simulink model "DC_Motor_Current_Control"  (R2024b)
settings: Solver=FixedStepDiscrete  StartTime=0.0  StopTime=15  FixedStep=0.001  RelTol=1e-3  EnableMultiTasking=on
undefined symbols (not defined in the file or in its folder): dspblkCoreblockFVToolHelper, gcbh
libraries: simulink x4, arduinolib x4, slpidlib x1
settings Model: ExtModeTrigDuration=2  Creator=BU  LastModifiedBy=BU
settings SolverCC: AutoInsertRateTranBlk=on
settings OptimizationCC: EnhancedBackFolding=on  PassReuseOutputArgsAs=Individual arguments  ZeroExternalMemoryAtStartup=off  ZeroInternalMemoryAtStartup=off  MaxStackSize=64  OptimizeBlockOrder=speed  DifferentSizesBufferReuse=on  OptimizationCustomize=off  EfficientTunableParamExpr=on
settings DebuggingCC: ParameterTunabilityLossMsg=error
settings HardwareCC: ProdBitPerInt=16  ProdBitPerPointer=16  ProdBitPerSizeT=16  ProdBitPerPtrDiffT=16  ProdLargestAtomicFloat=None  ProdWordSize=8  ProdHWDeviceType=Atmel->AVR  UseEmbeddedCoderFeatures=off  UseSimulinkCoderFeatures=off
settings SFSimCC: MATLABDynamicMemAlloc=off
settings RTWCC: Description=Embedded Coder  SystemTargetFile=ert.tlc  HardwareBoard=Arduino Mega 2560  TemplateMakefile=ert_default_tmf  Toolchain=Arduino AVR  BuildConfiguration=Faster Runs
settings CodeAppCC: ForceParamTrailComments=on  IgnoreCustomStorageClasses=off  OperatorAnnotations=on  SimulinkDataObjDesc=on  SFDataObjDesc=on  MangleLength=10  InsertBlockDesc=on
settings ERTTargetCC: SupportContinuousTime=on  SupportNonInlinedSFcns=on  SupportVariableSizeSignals=on  ExtModeTransport=3  ExtModeStaticAlloc=on  ExtModeAutomaticAllocSize=off  ExtModeStaticAllocSize=2048  ExtModeMexFile=ext_xcp  ExtModeIntrfLevel=Level2 - Open  InlinedParameterPlacement=Hierarchical

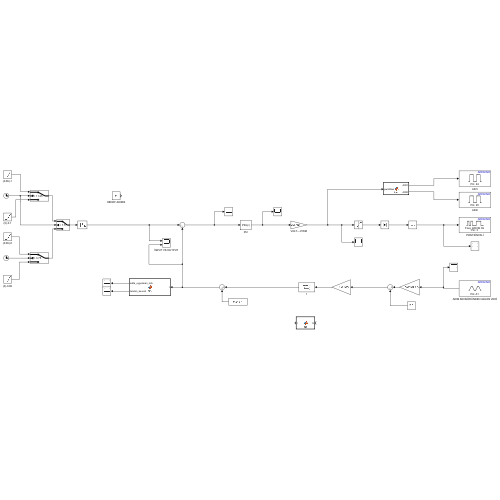
[thumbnail: Simulink's stored preview of the top-level diagram]
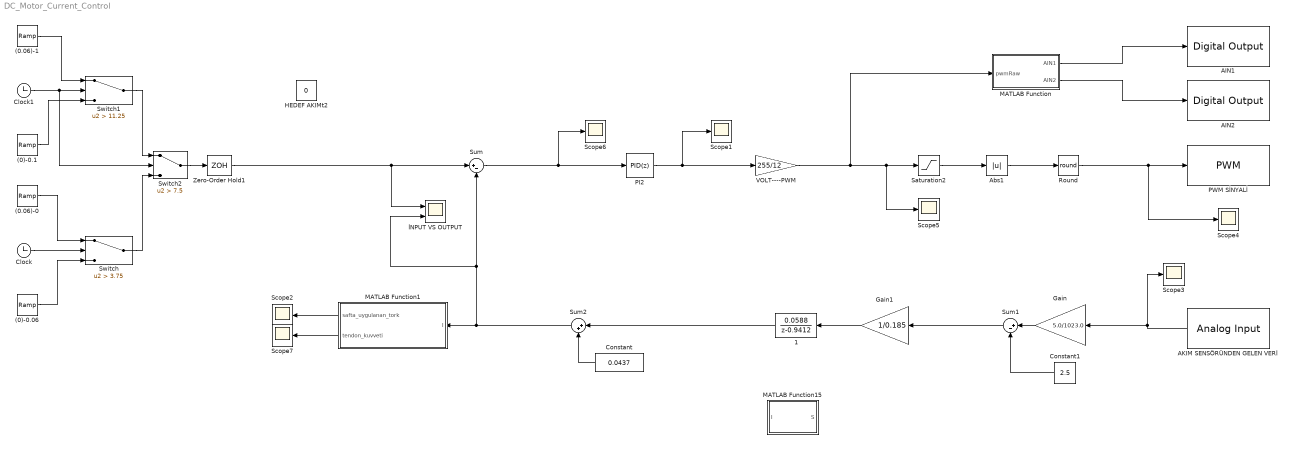
== system DC_Motor_Current_Control ==
  (0)-0.06 : simulink/Sources/Ramp  slope=0.013  start=0  InitialOutput=0
  (0)-0.1 : simulink/Sources/Ramp  slope=-0.013  start=7.5  InitialOutput=0
  (0.06)-0 : simulink/Sources/Ramp  slope=-0.013  start=3.75  InitialOutput=0.04875
  (0.06)-1 : simulink/Sources/Ramp  slope=0.013  start=11.25  InitialOutput=-0.04875
  1 : DiscreteTransferFcn  LoadFcn=dspblkCoreblockFVToolHelper(gcbh,'load');  Numerator=[0.0588]  Denominator=[1 -0.9412]
      settings: CopyFcn=dspblkCoreblockFVToolHelper(gcbh,'copy');  DeleteFcn=dspblkCoreblockFVToolHelper(gcbh,'close');  ModelCloseFcn=dspblkCoreblockFVToolHelper(gcbh,'close');  PreSaveFcn=dspblkCoreblockFVToolHelper(gcbh,'presave');  PostSaveFcn=dspblkCoreblockFVToolHelper(gcbh,'postsave');  CloseFcn=dspblkCoreblockFVToolHelper(gcbh,'close');
  AIN1 : arduinolib/Digital Output  pinNumber=24  Direction=output  blockPlatform=arduino
  AIN2 : arduinolib/Digital Output  pinNumber=25  Direction=output  blockPlatform=arduino
  AKIM SENSÖRÜNDEN GELEN VERİ : arduinolib/Analog Input  pinNumber=1  ReadResultsOnly=off  ConversionTriggerSource=Software  ExternalTriggerType=uint32( 0 )  OutputDataType=uint16  EnableConversionCompleteNotify=off  EnableOuputStatus=off  SampleTime=0.001  blockPlatform=arduino
  Abs1 : Abs  RndMeth=Round  SaturateOnIntegerOverflow=off
  Clock : Clock
  Clock1 : Clock
  Constant : Constant  Value=0.0437
  Constant1 : Constant  Value=2.5
  Gain : Gain  Gain=5.0/1023.0
  Gain1 : Gain  Gain=1/0.185
  HEDEF AKIMt2 : Constant  Value=0  VectorParams1D=off  SampleTime=0.001
  MATLAB Function : MATLAB Function  TreatAsAtomicUnit=on
  MATLAB Function1 : MATLAB Function  TreatAsAtomicUnit=on
  MATLAB Function15 : MATLAB Function  TreatAsAtomicUnit=on
  PI2 : slpidlib/PID Controller  Controller=PID  Form=Parallel  TimeDomain=Discrete-time  UseExternalTs=off  SampleTime=0.001  IntegratorMethod=Forward Euler  FilterMethod=Forward Euler  ControllerParametersSource=internal  P=21  I=900  UseKiTs=off  D=0.15  UseExternalDerivativeSource=off  N=100  UseFilter=off  TunerSelectOption=Transfer Function Based (PID Tuner App)  InitialConditionSource=internal  InitialConditionForIntegrator=0  InitialConditionForFilter=0  DifferentiatorICPrevScaledInput=0  ExternalReset=none  TrackingMode=off  Kt=1  LimitOutput=off  SatLimitsSource=internal  UpperSaturationLimit=inf  LowerSaturationLimit=-inf  LinearizeAsGain=on  AntiWindupMode=none  Kb=1  LimitIntegrator=off  UpperIntegratorSaturationLimit=inf  LowerIntegratorSaturationLimit=-inf  POutMin=[]  POutMax=[]  IOutMin=[]  IOutMax=[]  DOutMin=[]  DOutMax=[]  NOutMin=[]  NOutMax=[]  SumOutMin=[]  SumOutMax=[]  SaturationOutMin=[]  SaturationOutMax=[]  PParamMin=[]  PParamMax=[]  IParamMin=[]  IParamMax=[]  DParamMin=[]  DParamMax=[]  NParamMin=[]  NParamMax=[]  KbParamMin=[]  KbParamMax=[]  KtParamMin=[]  KtParamMax=[]  KbOutMin=[]  KbOutMax=[]  KtOutMin=[]  KtOutMax=[]  IntegratorOutMin=[]  IntegratorOutMax=[]  FilterOutMin=[]  FilterOutMax=[]  SumI1OutMin=[]  SumI1OutMax=[]  SumI2OutMin=[]  SumI2OutMax=[]  SumI3OutMin=[]  SumI3OutMax=[]  SumI4OutMin=[]  SumI4OutMax=[]  SumDOutMin=[]  SumDOutMax=[]  DifferentiatorOutMin=[]  DifferentiatorOutMax=[]  FilterDiffOutCoefMin=[]  FilterDiffOutCoefMax=[]  ReciprocalOutMin=[]  ReciprocalOutMax=[]  SumDenOutMin=[]  SumDenOutMax=[]  SumNumOutMin=[]  SumNumOutMax=[]  DivideOutMin=[]  DivideOutMax=[]  UdiffTsProdOutMin=[]  UdiffTsProdOutMax=[]  NTsProdOutMin=[]  NTsProdOutMax=[]  UintegralTsProdOutMin=[]  UintegralTsProdOutMax=[]  UngainTsProdOutMin=[]  UngainTsProdOutMax=[]  ClampingZeroOutDataTypeStr=Inherit: Inherit via back propagation  ClampingZeroOutMin=[]  ClampingZeroOutMax=[]  FilterDenConstantOutDataTypeStr=Inherit: Inherit via back propagation  FilterDenConstantOutMin=[]  FilterDenConstantOutMax=[]  PCopyOutDataTypeStr=Inherit: Inherit via back propagation  PCopyOutMin=[]  PCopyOutMax=[]  NCopyOutDataTypeStr=Inherit: Inherit via back propagation  NCopyOutMin=[]  NCopyOutMax=[]  IntegratorContinuousStateAttributes=''  IntegratorStateMustResolveToSignalObject=off  IntegratorRTWStateStorageClass=Auto  FilterContinuousStateAttributes=''  FilterStateMustResolveToSignalObject=off  FilterRTWStateStorageClass=Auto  ParallelPVariant=InternalParameters  IdealPVariant=Disabled  IVariant=InternalParameters  DVariant=InternalParameters  IntegratorVariant=Discrete  SatVariant=Disabled  AWVariant=Passthrough  PCopyVariant=Disabled  TRVariant=Disabled  FdbkBlocksVariant=Forward  IdealPFdbkVariant=Disabled  SatFdbkVariant=Disabled  DerivativeFilterVariant=Differentiator  NVariant=Passthrough  NCopyVariant=Disabled_SignalSpec  FilterICVariant=InternalICsDifferentiator  IntegratorICVariant=InternalICs  ExternalResetVariant=Disabled  TRSumVariant=Passthrough  SumFdbkVariant=Disabled  SumVariant=Sum_PID  TsampFilterVariant=InternalTs  TsampNgainVariant=Passthrough  TsampIntegralVariant=Disabled_SignalSpec  ExternalSaturationOutDataTypeStr=Inherit: Same as second input  DerivativeSourceVariant=ErrorSignal  PreIntVariant=InternalPreInt
  PWM SİNYALİ : arduinolib/PWM  pinNumber=3  frequencyType=Specify  desiredFrequency=490  achievableFrequency=489.9859
  Round : Rounding  Operator=round
  Saturation2 : Saturate  UpperLimit=255  LowerLimit=-255
  Scope{1..7} (7 alike) : Scope
  Sum : Sum  Inputs=|+-
  Sum1 : Sum  Inputs=|+-
  Sum2 : Sum  Inputs=|++
  Switch : Switch  Criteria=u2 > Threshold  Threshold=3.75  SaturateOnIntegerOverflow=off  InputSameDT=off
  Switch1 : Switch  Criteria=u2 > Threshold  Threshold=11.25  SaturateOnIntegerOverflow=off  InputSameDT=off
  Switch2 : Switch  Criteria=u2 > Threshold  Threshold=7.5  SaturateOnIntegerOverflow=off  InputSameDT=off
  VOLT----PWM : Gain  Gain=255/12
  Zero-Order Hold1 : ZeroOrderHold  SampleTime=0.001
  İNPUT VS OUTPUT : Scope  NumInputPorts=2
  wires:
  Abs1/1 -> Round/1
  Clock/1 -> Switch/2
  (0)-0.06/1 -> Switch/3
  Sum/1 -> PI2/1, Scope6/1
  Clock1/1 -> Switch1/2, Switch2/2
  PI2/1 -> VOLT----PWM/1, Scope1/1
  AKIM SENSÖRÜNDEN GELEN VERİ/1 -> Scope3/1, Gain/1
  Switch2/1 -> Zero-Order Hold1/1
  (0.06)-0/1 -> Switch/1
  (0)-0.1/1 -> Switch1/3
  Switch/1 -> Switch2/3
  VOLT----PWM/1 -> MATLAB Function/1(pwmRaw), Scope5/1, Saturation2/1
  Switch1/1 -> Switch2/1
  MATLAB Function/1(AIN1) -> AIN1/1
  MATLAB Function/2(AIN2) -> AIN2/1
  Saturation2/1 -> Abs1/1
  (0.06)-1/1 -> Switch1/1
  Round/1 -> Scope4/1, PWM SİNYALİ/1
  MATLAB Function1/2(tendon_kuvveti) -> Scope7/1
  MATLAB Function1/1(safta_uygulanan_tork) -> Scope2/1
  Gain/1 -> Sum1/1
  Constant1/1 -> Sum1/2
  Sum1/1 -> Gain1/1
  Gain1/1 -> 1/1
  1/1 -> Sum2/1
  Sum2/1 -> Sum/2, İNPUT VS OUTPUT/2, MATLAB Function1/1(I)
  Constant/1 -> Sum2/2
  Zero-Order Hold1/1 -> İNPUT VS OUTPUT/1, Sum/1

== matlab function DC_Motor_Current_Control/MATLAB Function1 ==
  data: I input; safta_uygulanan_tork output; tendon_kuvveti output
function [safta_uygulanan_tork, tendon_kuvveti] = fcn(I)

T = I*0.87;
tendon_kuvveti = T/(0.0125);
safta_uygulanan_tork = tendon_kuvveti*0.005;

end

== matlab function DC_Motor_Current_Control/MATLAB Function ==
  data: pwmRaw input; AIN1 output; AIN2 output
function [AIN1, AIN2] = fcn(pwmRaw)

if pwmRaw > 0
    AIN1=0;
    AIN2=1;
elseif pwmRaw <0 
    AIN1=1;
    AIN2=0;
else
    AIN1=0;
    AIN2=0;
end


end

== matlab function DC_Motor_Current_Control/MATLAB Function15 ==
  data: S input; I output
function I = fcn(S)

V = S*(5.0/1023.0);
I = (V-2.5)/0.185;

end
